simulink model "OMAP_ver_MIL10"  (R2018b)
settings: Solver=FixedStepDiscrete  StartTime=0.0  StopTime=10.0  FixedStep=0.01  RelTol=1e-3
undefined symbols (not defined in the file or in its folder): OMAP_Switch_EMS, OMAP_Switch_EPS, OMAP_Switch_ESC, OMAP_Switch_IC, OMAP_Switch_OTHER, TH_HMIClb_tiDgrdIconWarnHiDurT_C, TH_HMIClb_tiDgrdIconWarnLoDurT_C, TH_HMIClb_tiDgrdVocWarnDurT_C, TH_HMIClb_tiHndOffTxtWarnT_C, TH_HMIClb_tiHndOffVocWarnT_C, TH_HMIClb_tiSWALimFlgDetT_C, TH_HMIClb_tiTxtLimT_C
libraries: simulink x118
(part 1 of 9)
settings Model: Creator=许阁  LastModifiedBy=hj
settings OptimizationCC: BlockReduction=off  DefaultParameterBehavior=Inlined  DefaultUnderspecifiedDataType=single  EnhancedBackFolding=on  PassReuseOutputArgsAs=Individual arguments  ZeroExternalMemoryAtStartup=off  ZeroInternalMemoryAtStartup=off  OptimizeBlockOrder=speed  DifferentSizesBufferReuse=on  OptimizationCustomize=off
settings DebuggingCC: ParameterTunabilityLossMsg=error
settings SFSimCC: MATLABDynamicMemAlloc=off
settings RTWCC: SystemTargetFile=autosar.tlc  GenCodeOnly=on  TemplateMakefile=ert_default_tmf  Description=AUTOSAR  GenerateReport=on  IncludeHyperlinkInReport=on  LaunchReport=on  GenerateTraceInfo=on  GenerateTraceReport=on  GenerateTraceReportSl=on  GenerateTraceReportSf=on  GenerateTraceReportEml=on  GenerateCodeMetricsReport=on
settings CodeAppCC: ForceParamTrailComments=on  IgnoreCustomStorageClasses=off  OperatorAnnotations=on  SimulinkDataObjDesc=on  SFDataObjDesc=on  InsertBlockDesc=on
settings STFCustomTargetCC: TargetLangStandard=C99 (ISO)  MultiwordLength=256  ParMdlRefBuildCompliant=on  CompOptLevelCompliant=on  IncludeMdlTerminateFcn=off  CombineOutputUpdateFcns=on  SuppressErrorStatus=on  ERTCustomFileBanners=on  SupportNonFinite=off  SupportComplex=off  SupportContinuousTime=off  SupportNonInlinedSFcns=off  RemoveResetFunc=on  MATLABClassNameForMDSCustomization=Simulink.SoftwareTarget.ERTCustomization  AutosarCompliant=on  UseToolchainInfoCompliant=on  LookupTableObjectStructAxisOrder=2,1,3,4,...  LUTObjectStructOrderEvenSpacing=Size,Table,Breakpoints  SystemTargetFile=autosar.tlc
settings ERTTargetCC: TargetLangStandard=C99 (ISO)  ConcurrentExecutionCompliant=off  IncludeMdlTerminateFcn=off  SuppressErrorStatus=on  SupportNonFinite=off  SupportComplex=off  ModelStepFunctionPrototypeControlCompliant=off  CPPClassGenCompliant=off  AutosarCompliant=on  LookupTableObjectStructAxisOrder=2,1,3,4,...  LUTObjectStructOrderEvenSpacing=Size,Table,Breakpoints  GenerateASAP2=on  InlinedParameterPlacement=NonHierarchical  ERTCustomFileTemplate=example_file_process.tlc

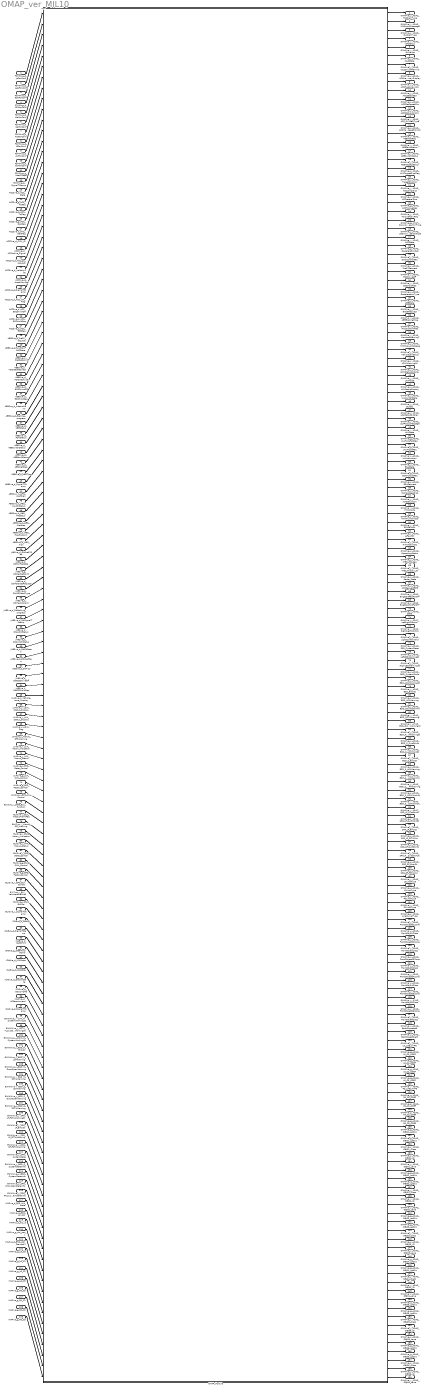
== system OMAP_ver_MIL10 ==
  FDMMve_d_JaFcnConf : Inport  OutDataTypeStr=UInt16  PortDimensions=1
  FDMMve_d_AebFcnConf : Inport  Port=2  OutDataTypeStr=UInt16  PortDimensions=1
  FDMMve_d_EsaFcnConf : Inport  Port=3  OutDataTypeStr=UInt16  PortDimensions=1
  FDMMve_d_ElkFcnConf : Inport  Port=4  OutDataTypeStr=UInt16  PortDimensions=1
  FDMMve_d_LkaFcnConf : Inport  Port=5  OutDataTypeStr=UInt16  PortDimensions=1
  FDMMve_d_IcaFcnConf : Inport  Port=6  OutDataTypeStr=UInt16  PortDimensions=1
  FDMMve_d_AccFcnConf : Inport  Port=7  OutDataTypeStr=UInt16  PortDimensions=1
  FDMMve_d_LfFcnConf : Inport  Port=8  OutDataTypeStr=UInt16  PortDimensions=1
  FDMMve_d_AlcFcnConf : Inport  Port=9  OutDataTypeStr=UInt16  PortDimensions=1
  FDMMve_d_EwFcnConf : Inport  Port=10  OutDataTypeStr=UInt16  PortDimensions=1
  FDMMve_g_Adas2Fapa : Inport  Port=11  OutDataTypeStr=UInt32  PortDimensions=1
  FDMMve_d_SignalTStamp : Inport  Port=12  OutDataTypeStr=UInt16  PortDimensions=1
  ACCSve_d_ACC_State : Inport  Port=13  OutDataTypeStr=UInt16  PortDimensions=1
  ACCSve_g_ACC_TqReq : Inport  Port=14  OutDataTypeStr=T_M_Nm_Float32  PortDimensions=1
  ACCSve_d_ACC_TqFlag : Inport  Port=15  OutDataTypeStr=UInt16  PortDimensions=1
  ACCSve_g_ACC_DecReq : Inport  Port=16  OutDataTypeStr=T_M_Nm_Float32  PortDimensions=1
  ACCSve_d_ACC_DecFlag : Inport  Port=17  OutDataTypeStr=UInt16  PortDimensions=1
  ACCSve_d_CIPV_ID : Inport  Port=18  OutDataTypeStr=UInt16  PortDimensions=1
  ACCSve_d_ACCActive_Signal : Inport  Port=19  OutDataTypeStr=UInt16  PortDimensions=1
  ACCSve_d_ACC_go_request : Inport  Port=20  OutDataTypeStr=UInt16  PortDimensions=1
  ACCSve_d_VelocitySet : Inport  Port=21  OutDataTypeStr=UInt16  PortDimensions=1
  ACCSve_d_HeadWaySet : Inport  Port=22  OutDataTypeStr=UInt16  PortDimensions=1
  ACCSve_d_SignalTStamp : Inport  Port=23  OutDataTypeStr=UInt16  PortDimensions=1
  ACCSve_d_ACC_ICA_Flag : Inport  Port=24  OutDataTypeStr=UInt16  PortDimensions=1
  ACCSve_d_ACC_ESCDriveOff : Inport  Port=25  OutDataTypeStr=UInt16  PortDimensions=1
  ACCSve_d_ACC_ESCHoldReq : Inport  Port=26  OutDataTypeStr=UInt16  PortDimensions=1
  ACCSve_d_ACC_EPBReq : Inport  Port=27  OutDataTypeStr=UInt16  PortDimensions=1
  AEBSve_d_Prefill_request : Inport  Port=28  OutDataTypeStr=UInt16  PortDimensions=1
  AEBSve_d_functionFARCState : Inport  Port=29  OutDataTypeStr=UInt16  PortDimensions=1
  AEBSve_g_DecSetpoint : Inport  Port=30  OutDataTypeStr=T_M_Nm_Float32  PortDimensions=1
  AEBSve_d_MDDdecRequest : Inport  Port=31  OutDataTypeStr=UInt16  PortDimensions=1
  AEBSve_d_MDDdecType : Inport  Port=32  OutDataTypeStr=UInt16  PortDimensions=1
  AEBSve_d_ESCDriveOff : Inport  Port=33  OutDataTypeStr=UInt16  PortDimensions=1
  AEBSve_d_ESCHoldReq : Inport  Port=34  OutDataTypeStr=UInt16  PortDimensions=1
  AEBSve_d_HapticAlarm : Inport  Port=35  OutDataTypeStr=UInt16  PortDimensions=1
  AEBSve_d_Braking_progress : Inport  Port=36  OutDataTypeStr=UInt16  PortDimensions=1
  AEBSve_d_AEBStatus : Inport  Port=37  OutDataTypeStr=UInt16  PortDimensions=1
  AEBSve_d_FCWStatus : Inport  Port=38  OutDataTypeStr=UInt16  PortDimensions=1
  AEBSve_d_AEBSwitchStatus : Inport  Port=39  OutDataTypeStr=UInt16  PortDimensions=1
  AEBSve_d_AEBFaultStatus : Inport  Port=40  OutDataTypeStr=UInt16  PortDimensions=1
  AEBSve_d_AEBAlertReq : Inport  Port=41  OutDataTypeStr=UInt16  PortDimensions=1
  AEBSve_d_AEBTips : Inport  Port=42  OutDataTypeStr=UInt16  PortDimensions=1
  AEBSve_d_SignalTStamp : Inport  Port=43  OutDataTypeStr=UInt16  PortDimensions=1
  AEBSve_d_JABS_AlertSign : Inport  Port=44  OutDataTypeStr=UInt16  PortDimensions=1
  AEBSve_d_JABS_SwitchStatus : Inport  Port=45  OutDataTypeStr=UInt16  PortDimensions=1
  AEBSve_d_JABS_FltStatus : Inport  Port=46  OutDataTypeStr=UInt16  PortDimensions=1
  AEBSve_d_JABS_AlertReq : Inport  Port=47  OutDataTypeStr=UInt16  PortDimensions=1
  AEBSve_d_JABS_HapticAlarm : Inport  Port=48  OutDataTypeStr=UInt16  PortDimensions=1
  AEBSve_d_JABS_Tips : Inport  Port=49  OutDataTypeStr=UInt16  PortDimensions=1
  JABSve_d_DbPrefillReq : Inport  Port=50  OutDataTypeStr=UInt16  PortDimensions=1
  JABSve_d_DbFunFARCSta : Inport  Port=51  OutDataTypeStr=UInt16  PortDimensions=1
  JABSve_g_DbDecSetpoint : Inport  Port=52  OutDataTypeStr=T_M_Nm_Float32  PortDimensions=1
  JABSve_d_DbMDDdecRequest : Inport  Port=53  OutDataTypeStr=UInt16  PortDimensions=1
  JABSve_d_DbMDDdecType : Inport  Port=54  OutDataTypeStr=UInt16  PortDimensions=1
  JABSve_d_DbHapticAlarm : Inport  Port=55  OutDataTypeStr=UInt16  PortDimensions=1
  JABSve_d_DbBraking_progress : Inport  Port=56  OutDataTypeStr=UInt16  PortDimensions=1
  JABSve_d_DbSignalTStamp : Inport  Port=57  OutDataTypeStr=UInt16  PortDimensions=1
  JABSve_d_DbJACWStatus : Inport  Port=58  OutDataTypeStr=UInt16  PortDimensions=1
  JABSve_d_DbSwitchStatus : Inport  Port=59  OutDataTypeStr=UInt16  PortDimensions=1
  JABSve_d_DbFltStatus : Inport  Port=60  OutDataTypeStr=UInt16  PortDimensions=1
  JABSve_d_DbAlertReq : Inport  Port=61  OutDataTypeStr=UInt16  PortDimensions=1
  JABSve_d_DbTips : Inport  Port=62  OutDataTypeStr=UInt16  PortDimensions=1
  JABSve_d_DbESCDriveOff : Inport  Port=63  OutDataTypeStr=UInt16  PortDimensions=1
  JABSve_d_DbESCHoldReq : Inport  Port=64  OutDataTypeStr=UInt16  PortDimensions=1
  LKASve_y_Vehicle_Lane_Display : Inport  Port=65  OutDataTypeStr=UInt8  PortDimensions=1
  LKASve_y_LDW_Status_Display : Inport  Port=66  OutDataTypeStr=UInt8  PortDimensions=1
  LKASve_y_LKA_Status_Display : Inport  Port=67  OutDataTypeStr=UInt8  PortDimensions=1
  LKASve_y_LDW_Flag : Inport  Port=68  OutDataTypeStr=UInt8  PortDimensions=1
  LKASve_y_Hands_Off_Warning : Inport  Port=69  OutDataTypeStr=UInt8  PortDimensions=1
  LKASve_y_LKA_Action_Indication : Inport  Port=70  OutDataTypeStr=UInt8  PortDimensions=1
  LKASve_y_HMI_Popup_Status : Inport  Port=71  OutDataTypeStr=UInt8  PortDimensions=1
  LKASve_y_EPS_State_Control : Inport  Port=72  OutDataTypeStr=UInt8  PortDimensions=1
  LKASve_g_LKA_SWA_Control : Inport  Port=73  OutDataTypeStr=T_M_Nm_Float32  PortDimensions=1
  LKASve_g_EPS_Factor_Control : Inport  Port=74  OutDataTypeStr=T_M_Nm_Float32  PortDimensions=1
  LKASve_y_EPS_LKA_Control : Inport  Port=75  OutDataTypeStr=UInt8  PortDimensions=1
  ELKSve_y_state_ELK_function : Inport  Port=76  OutDataTypeStr=UInt8  PortDimensions=1
  ELKSve_y_ELK_HapticAlarmReq : Inport  Port=77  OutDataTypeStr=UInt8  PortDimensions=1
  ELKSve_y_Hands_Off_Warning : Inport  Port=78  OutDataTypeStr=UInt8  PortDimensions=1
  ELKSve_y_ELK_Action_Indication : Inport  Port=79  OutDataTypeStr=UInt8  PortDimensions=1
  ELKSve_y_HMI_Popup_Status : Inport  Port=80  OutDataTypeStr=UInt8  PortDimensions=1
  ELKSve_y_EPS_State_Control : Inport  Port=81  OutDataTypeStr=UInt8  PortDimensions=1
  ELKSve_g_ELK_SWA_Control : Inport  Port=82  OutDataTypeStr=T_M_Nm_Float32  PortDimensions=1
  ELKSve_g_EPS_Factor_Control : Inport  Port=83  OutDataTypeStr=T_M_Nm_Float32  PortDimensions=1
  ELKSve_y_EPS_ELK_Control : Inport  Port=84  OutDataTypeStr=UInt8  PortDimensions=1
  ELKSve_y_ELK_VehicleLaneDisp : Inport  Port=85  OutDataTypeStr=UInt8  PortDimensions=1
  ELKSve_y_ELK_ELKSts : Inport  Port=86  OutDataTypeStr=UInt8  PortDimensions=1
  ELKSve_y_SignalTStamp : Inport  Port=87  OutDataTypeStr=UInt8  PortDimensions=1
  ICABva_d_PathQI : Inport  Port=88  OutDataTypeStr=UInt16  PortDimensions=6
  ICABve_d_SignalTStamp : Inport  Port=89  OutDataTypeStr=UInt16  PortDimensions=1
  ICABva_d_ICAB2HMI : Inport  Port=90  OutDataTypeStr=UInt16  PortDimensions=20
  ICABve_g_SteerAngleCmd : Inport  Port=91  OutDataTypeStr=T_M_Nm_Float32  PortDimensions=1
  ICABve_d_ICAMode : Inport  Port=92  OutDataTypeStr=UInt16  PortDimensions=1
  ICABve_d_ICAState : Inport  Port=93  OutDataTypeStr=UInt16  PortDimensions=1
  ICADva_d_DecionState : Inport  Port=94  OutDataTypeStr=UInt16  PortDimensions=10
  ICADva_d_DecionCMD : Inport  Port=95  OutDataTypeStr=UInt16  PortDimensions=10
  ICADva_d_LCRecommend : Inport  Port=96  OutDataTypeStr=UInt16  PortDimensions=10
  ICADve_d_SignalTStamp : Inport  Port=97  OutDataTypeStr=UInt16  PortDimensions=1
  EWWWve_y_LCW_M_SystemWorkingSt : Inport  Port=98  OutDataTypeStr=UInt8  PortDimensions=1
  EWWWve_y_RCTA_M_SystemWorkingSt : Inport  Port=99  OutDataTypeStr=UInt8  PortDimensions=1
  EWWWve_y_DOW_M_SystemWorkingSt : Inport  Port=100  OutDataTypeStr=UInt8  PortDimensions=1
  EWWWve_y_BSD_M_ErrorSt : Inport  Port=101  OutDataTypeStr=UInt8  PortDimensions=1
  EWWWve_y_BSD_M_LCAWarning : Inport  Port=102  OutDataTypeStr=UInt8  PortDimensions=1
  EWWWve_y_BSD_M_DoorOpenWarning : Inport  Port=103  OutDataTypeStr=UInt8  PortDimensions=1
  EWWWve_y_BSD_M_RCTAWarning : Inport  Port=104  OutDataTypeStr=UInt8  PortDimensions=1
  EWWWve_y_BSD_S_LCAWarning : Inport  Port=105  OutDataTypeStr=UInt8  PortDimensions=1
  EWWWve_y_BSD_S_DoorOpenWarning : Inport  Port=106  OutDataTypeStr=UInt8  PortDimensions=1
  EWWWve_y_BSD_S_RCTAWarning : Inport  Port=107  OutDataTypeStr=UInt8  PortDimensions=1
  EWWWve_y_SRR_LF_FCTAWorkingSt : Inport  Port=108  OutDataTypeStr=UInt8  PortDimensions=1
  EWWWve_y_SRR_LF_ErrorSt : Inport  Port=109  OutDataTypeStr=UInt8  PortDimensions=1
  EWWWve_y_SRR_LF_FCTAWarning : Inport  Port=110  OutDataTypeStr=UInt8  PortDimensions=1
  EWWWve_y_SRR_RF_FCTAWarning : Inport  Port=111  OutDataTypeStr=UInt8  PortDimensions=1
  EWWWve_y_SRR_SystemState : Inport  Port=112  OutDataTypeStr=UInt8  PortDimensions=1
  EWWWve_y_BSD_S_SystemStateInfo : Inport  Port=113  OutDataTypeStr=UInt8  PortDimensions=1
  EWWWve_y_BSD_SystemStateInfo : Inport  Port=114  OutDataTypeStr=UInt8  PortDimensions=1
  EWWWve_y_SRR_LF_SystemStateInfo : Inport  Port=115  OutDataTypeStr=UInt8  PortDimensions=1
  EWWWve_y_SRR_RF_SystemStateInfo : Inport  Port=116  OutDataTypeStr=UInt8  PortDimensions=1
  IMAPve_d_EPS_LKA_State : Inport  Port=117  OutDataTypeStr=UInt16  PortDimensions=1
  IMAPve_g_ESC_LonAcc : Inport  Port=118  OutDataTypeStr=T_M_Nm_Float32  PortDimensions=1
  IMAPva_d_obj_id : Inport  Port=119  OutDataTypeStr=UInt16  PortDimensions=40
  IMAPva_g_obj_pos_x : Inport  Port=120  OutDataTypeStr=T_M_Nm_Float32  PortDimensions=40
  IMAPve_d_ESC_Veh_Standstill : Inport  Port=121  OutDataTypeStr=UInt16  PortDimensions=1
  IMAPve_g_L0_C0 : Inport  Port=122  OutDataTypeStr=T_M_Nm_Float32  PortDimensions=1
  IMAPve_g_L0_C1 : Inport  Port=123  OutDataTypeStr=T_M_Nm_Float32  PortDimensions=1
  IMAPve_g_L0_C2 : Inport  Port=124  OutDataTypeStr=T_M_Nm_Float32  PortDimensions=1
  IMAPve_g_L0_C3 : Inport  Port=125  OutDataTypeStr=T_M_Nm_Float32  PortDimensions=1
  IMAPve_g_R0_C0 : Inport  Port=126  OutDataTypeStr=T_M_Nm_Float32  PortDimensions=1
  IMAPve_g_R0_C1 : Inport  Port=127  OutDataTypeStr=T_M_Nm_Float32  PortDimensions=1
  IMAPve_g_R0_C2 : Inport  Port=128  OutDataTypeStr=T_M_Nm_Float32  PortDimensions=1
  IMAPve_g_R0_C3 : Inport  Port=129  OutDataTypeStr=T_M_Nm_Float32  PortDimensions=1
  OMAP_Module : Subsystem  TreatAsAtomicUnit=on
  OMAPve_y_ADAS_TSRSignType : Outport  OutDataTypeStr=UInt8  PortDimensions=1
  OMAPve_y_ADAS_ISAPopupMessage : Outport  Port=2  OutDataTypeStr=UInt8  PortDimensions=1
  OMAPve_y_ADAS_ISASignType : Outport  Port=3  OutDataTypeStr=UInt8  PortDimensions=1
  OMAPve_y_ADAS_ISAStatus : Outport  Port=4  OutDataTypeStr=UInt8  PortDimensions=1
  OMAPve_y_ADAS_ISAValue : Outport  Port=5  OutDataTypeStr=UInt8  PortDimensions=1
  OMAPve_y_ADAS_ISLCState : Outport  Port=6  OutDataTypeStr=UInt8  PortDimensions=1
  OMAPve_y_ADAS_ISLCDriverRemind : Outport  Port=7  OutDataTypeStr=UInt8  PortDimensions=1
  OMAPve_y_ADAS_ACCHeadwayDisplay : Outport  Port=8  OutDataTypeStr=UInt8  PortDimensions=1
  OMAPve_y_ADAS_ACCHeadwayIcon : Outport  Port=9  OutDataTypeStr=UInt8  PortDimensions=1
  OMAPve_y_ADAS_ACCSetSpeed : Outport  Port=10  OutDataTypeStr=UInt8  PortDimensions=1
  OMAPve_y_ADAS_ACCSetSpeedDis : Outport  Port=11  OutDataTypeStr=UInt8  PortDimensions=1
  OMAPve_y_ADAS_ACCStatusIconDis : Outport  Port=12  OutDataTypeStr=UInt8  PortDimensions=1
  OMAPve_y_ADAS_ACC_RVVReqType : Outport  Port=13  OutDataTypeStr=UInt8  PortDimensions=1
  OMAPve_y_ADAS_ACCMessagePrompt : Outport  Port=14  OutDataTypeStr=UInt8  PortDimensions=1
  OMAPve_y_ADAS_AEBAlertReq : Outport  Port=15  OutDataTypeStr=UInt8  PortDimensions=1
  OMAPve_y_ADAS_AEBFaultStatus : Outport  Port=16  OutDataTypeStr=UInt8  PortDimensions=1
  OMAPve_y_ADAS_AEBSwitchStatus : Outport  Port=17  OutDataTypeStr=UInt8  PortDimensions=1
  OMAPve_y_ADAS_AEBMassageDisp : Outport  Port=18  OutDataTypeStr=UInt8  PortDimensions=1
  OMAPve_y_ADAS_HMITargetDispFlag : Outport  Port=19  OutDataTypeStr=UInt8  PortDimensions=1
  OMAPve_y_ADAS_TargetPosition : Outport  Port=20  OutDataTypeStr=UInt8  PortDimensions=1
  OMAPve_y_ADAS_ACCLongiDist : Outport  Port=21  OutDataTypeStr=UInt8  PortDimensions=1
  OMAPve_y_ADAS_ACCLateralDist : Outport  Port=22  OutDataTypeStr=SInt8  PortDimensions=1
  OMAPve_g_ADAS_ACCTorqueReq : Outport  Port=23  OutDataTypeStr=T_M_Nm_Float32  PortDimensions=1
  OMAPve_y_ADAS_TorqueActivReq : Outport  Port=24  OutDataTypeStr=UInt8  PortDimensions=1
  OMAPve_g_ADAS_DownorUpGearMinTime : Outport  Port=25  OutDataTypeStr=T_M_Nm_Float32  PortDimensions=1
  OMAPve_y_ADAS_UpDownGearChange : Outport  Port=26  OutDataTypeStr=UInt8  PortDimensions=1
  OMAPve_y_ADAS_ACCState : Outport  Port=27  OutDataTypeStr=UInt8  PortDimensions=1
  OMAPve_g_ADAS_DecelerationSet : Outport  Port=28  OutDataTypeStr=T_M_Nm_Float32  PortDimensions=1
  OMAPve_y_ADAS_DeclControlReq : Outport  Port=29  OutDataTypeStr=UInt8  PortDimensions=1
  OMAPve_y_ADAS_PrefillRequest : Outport  Port=30  OutDataTypeStr=UInt8  PortDimensions=1
  OMAPve_y_ADAS_ESCDriveOff : Outport  Port=31  OutDataTypeStr=UInt8  PortDimensions=1
  OMAPve_y_ADAS_ESCHoldReq : Outport  Port=32  OutDataTypeStr=UInt8  PortDimensions=1
  OMAPve_y_ADAS_DecelerationType : Outport  Port=33  OutDataTypeStr=UInt8  PortDimensions=1
  OMAPve_y_ADAS_AEBState : Outport  Port=34  OutDataTypeStr=UInt8  PortDimensions=1
  OMAPve_y_ADAS_BrakeRequest : Outport  Port=35  OutDataTypeStr=UInt8  PortDimensions=1
  OMAPve_y_ADAS_AEBBrakingProg : Outport  Port=36  OutDataTypeStr=UInt8  PortDimensions=1
  OMAPve_y_ADAS_HapticAlarmReq : Outport  Port=37  OutDataTypeStr=UInt8  PortDimensions=1
  OMAPve_y_ADAS_Handsoffwarning : Outport  Port=38  OutDataTypeStr=UInt8  PortDimensions=1
  OMAPve_y_ADAS_HMIPopupMassage : Outport  Port=39  OutDataTypeStr=UInt8  PortDimensions=1
  OMAPve_y_ADAS_VehicleLaneDisp : Outport  Port=40  OutDataTypeStr=UInt8  PortDimensions=1
  OMAPve_y_ADAS_LDWWarningSt : Outport  Port=41  OutDataTypeStr=UInt8  PortDimensions=1
  OMAPve_y_ADAS_LDWStatusDisplay : Outport  Port=42  OutDataTypeStr=UInt8  PortDimensions=1
  OMAPve_y_ADAS_LKAMode : Outport  Port=43  OutDataTypeStr=UInt8  PortDimensions=1
  OMAPve_y_ADAS_LKAStatusDisplay : Outport  Port=44  OutDataTypeStr=UInt8  PortDimensions=1
  OMAPve_y_ADAS_LKASwitchState : Outport  Port=45  OutDataTypeStr=UInt8  PortDimensions=1
  OMAPve_y_ADAS_ELKSts : Outport  Port=46  OutDataTypeStr=UInt8  PortDimensions=1
  OMAPve_y_ADAS_LCAStatusDisplay : Outport  Port=47  OutDataTypeStr=UInt8  PortDimensions=1
  OMAPve_y_ADAS_LCAPopupMessage : Outport  Port=48  OutDataTypeStr=UInt8  PortDimensions=1
  OMAPve_y_ADAS_LKAState : Outport  Port=49  OutDataTypeStr=UInt8  PortDimensions=1
  OMAPve_g_ADAS_LKATorqFactReq : Outport  Port=50  OutDataTypeStr=T_M_Nm_Float32  PortDimensions=1
  OMAPve_g_ADAS_LKAAngleReq : Outport  Port=51  OutDataTypeStr=T_M_Nm_Float32  PortDimensions=1
  OMAPve_y_ADAS_LKAActivation : Outport  Port=52  OutDataTypeStr=UInt8  PortDimensions=1
  OMAPve_y_ADAS_ESAState : Outport  Port=53  OutDataTypeStr=UInt8  PortDimensions=1
  OMAPve_g_ADAS_ESATorqueReq : Outport  Port=54  OutDataTypeStr=T_M_Nm_Float32  PortDimensions=1
  OMAPve_y_ADAS_ESARequest : Outport  Port=55  OutDataTypeStr=UInt8  PortDimensions=1
  OMAPve_y_ADAS_ICAMassageDisp : Outport  Port=56  OutDataTypeStr=UInt8  PortDimensions=1
  OMAPve_y_ADAS_ICAStatusIcon : Outport  Port=57  OutDataTypeStr=UInt8  PortDimensions=1
  OMAPve_y_ADAS_HWAMode : Outport  Port=58  OutDataTypeStr=UInt8  PortDimensions=1
  OMAPve_y_ADAS_HWATurnOnIdctr : Outport  Port=59  OutDataTypeStr=UInt8  PortDimensions=1
  OMAPve_y_ADAS_ESAFaultSt : Outport  Port=60  OutDataTypeStr=UInt8  PortDimensions=1
  OMAPve_y_ADAS_JAFaultSt : Outport  Port=61  OutDataTypeStr=UInt8  PortDimensions=1
  OMAPve_y_ADAS_HWAActionSts : Outport  Port=62  OutDataTypeStr=UInt8  PortDimensions=1
  OMAPve_y_ADAS_OperatingStatus : Outport  Port=63  OutDataTypeStr=UInt8  PortDimensions=1
  OMAPve_y_ADAS_IHBC_HB_Req : Outport  Port=64  OutDataTypeStr=UInt8  PortDimensions=1
  OMAPve_y_ADAS_IHBC_Fuction_St : Outport  Port=65  OutDataTypeStr=UInt8  PortDimensions=1
  OMAPve_y_ADAS_Radar_State : Outport  Port=66  OutDataTypeStr=UInt8  PortDimensions=1
  OMAPve_y_ADAS_ACCRequestEPB : Outport  Port=67  OutDataTypeStr=UInt8  PortDimensions=1
  OMAPve_y_ADAS_EngStartReqForSTT : Outport  Port=68  OutDataTypeStr=UInt8  PortDimensions=1
  OMAPve_y_ADAS_EngStopPmtForSTT : Outport  Port=69  OutDataTypeStr=UInt8  PortDimensions=1
  OMAPve_y_ADAS_State : Outport  Port=70  OutDataTypeStr=UInt8  PortDimensions=1
  OMAPve_y_ADAS_LetfLigthControl : Outport  Port=71  OutDataTypeStr=UInt8  PortDimensions=1
  OMAPve_y_ADAS_RightLigthControl : Outport  Port=72  OutDataTypeStr=UInt8  PortDimensions=1
  OMAPve_y_ADAS_LightControlValid : Outport  Port=73  OutDataTypeStr=UInt8  PortDimensions=1
  OMAPve_y_ADAS_SRR_SystemState : Outport  Port=74  OutDataTypeStr=UInt8  PortDimensions=1
  OMAPve_y_ADAS_LeftLEDWarningSt : Outport  Port=75  OutDataTypeStr=UInt8  PortDimensions=1
  OMAPve_y_ADAS_RighrLEDWarningSt : Outport  Port=76  OutDataTypeStr=UInt8  PortDimensions=1
  OMAPve_y_ADAS_BSD_SystemStInfo : Outport  Port=77  OutDataTypeStr=UInt8  PortDimensions=1
  OMAPve_y_ADAS_BSD_LCWWorkingSt : Outport  Port=78  OutDataTypeStr=UInt8  PortDimensions=1
  OMAPve_y_ADAS_BSD_ErrorSt : Outport  Port=79  OutDataTypeStr=UInt8  PortDimensions=1
  OMAPve_y_ADAS_BSD_LCAWarning : Outport  Port=80  OutDataTypeStr=UInt8  PortDimensions=1
  OMAPve_y_ADAS_BSD_DoorOpenWrn : Outport  Port=81  OutDataTypeStr=UInt8  PortDimensions=1
  OMAPve_y_ADAS_BSD_RCTAWarning : Outport  Port=82  OutDataTypeStr=UInt8  PortDimensions=1
  OMAPve_y_ADAS_BSD_DOWWorkingSt : Outport  Port=83  OutDataTypeStr=UInt8  PortDimensions=1
  OMAPve_y_ADAS_BSD_RCTAWorkingSt : Outport  Port=84  OutDataTypeStr=UInt8  PortDimensions=1
  OMAPve_y_ADAS_BSD_S_SystStInfo : Outport  Port=85  OutDataTypeStr=UInt8  PortDimensions=1
  OMAPve_y_ADAS_BSD_S_LCWWorkSt : Outport  Port=86  OutDataTypeStr=UInt8  PortDimensions=1
  OMAPve_y_ADAS_BSD_S_ErrorSt : Outport  Port=87  OutDataTypeStr=UInt8  PortDimensions=1
  OMAPve_y_ADAS_BSD_S_LCAWarning : Outport  Port=88  OutDataTypeStr=UInt8  PortDimensions=1
  OMAPve_y_ADAS_BSD_S_DoorOpenWrn : Outport  Port=89  OutDataTypeStr=UInt8  PortDimensions=1
  OMAPve_y_ADAS_BSD_S_RCTAWarning : Outport  Port=90  OutDataTypeStr=UInt8  PortDimensions=1
  OMAPve_y_ADAS_BSD_S_DOWWorkSt : Outport  Port=91  OutDataTypeStr=UInt8  PortDimensions=1
  OMAPve_y_ADAS_BSD_S_RCTAWorkSt : Outport  Port=92  OutDataTypeStr=UInt8  PortDimensions=1
  OMAPve_y_ADAS_SRR_LF_SystStInfo : Outport  Port=93  OutDataTypeStr=UInt8  PortDimensions=1
  OMAPve_y_ADAS_SRR_LF_SystWorkSt : Outport  Port=94  OutDataTypeStr=UInt8  PortDimensions=1
  OMAPve_y_ADAS_SRR_LF_ErrorSt : Outport  Port=95  OutDataTypeStr=UInt8  PortDimensions=1
  OMAPve_y_ADAS_SRR_LF_FCTAWrn : Outport  Port=96  OutDataTypeStr=UInt8  PortDimensions=1
  OMAPve_y_ADAS_SRR_RF_SystStInfo : Outport  Port=97  OutDataTypeStr=UInt8  PortDimensions=1
  OMAPve_y_ADAS_SRR_RF_SystWorkSt : Outport  Port=98  OutDataTypeStr=UInt8  PortDimensions=1
  OMAPve_y_ADAS_SRR_RF_ErrorSt : Outport  Port=99  OutDataTypeStr=UInt8  PortDimensions=1
  OMAPve_y_ADAS_SRR_RF_FCTAWrn : Outport  Port=100  OutDataTypeStr=UInt8  PortDimensions=1
  OMAPve_y_ADAS_L0LineType : Outport  Port=101  OutDataTypeStr=UInt8  PortDimensions=1
  OMAPve_y_ADAS_L1LineType : Outport  Port=102  OutDataTypeStr=UInt8  PortDimensions=1
  OMAPve_y_ADAS_R0LineType : Outport  Port=103  OutDataTypeStr=UInt8  PortDimensions=1
  OMAPve_y_ADAS_R1LineType : Outport  Port=104  OutDataTypeStr=UInt8  PortDimensions=1
  OMAPve_y_ADAS_LineCurveType : Outport  Port=105  OutDataTypeStr=UInt8  PortDimensions=1
  OMAPve_y_ADAS_FrontObject01Zone : Outport  Port=106  OutDataTypeStr=UInt8  PortDimensions=1
  OMAPve_y_ADAS_FrontObj01Class : Outport  Port=107  OutDataTypeStr=UInt8  PortDimensions=1
  OMAPve_y_ADAS_FrontObject02Zone : Outport  Port=108  OutDataTypeStr=UInt8  PortDimensions=1
  OMAPve_y_ADAS_FrontObj02Class : Outport  Port=109  OutDataTypeStr=UInt8  PortDimensions=1
  OMAPve_y_ADAS_FrontObject03Zone : Outport  Port=110  OutDataTypeStr=UInt8  PortDimensions=1
  OMAPve_y_ADAS_FrontObj03Class : Outport  Port=111  OutDataTypeStr=UInt8  PortDimensions=1
  OMAPve_y_ADAS_FrontObject04Zone : Outport  Port=112  OutDataTypeStr=UInt8  PortDimensions=1
  OMAPve_y_ADAS_FrontObj04Class : Outport  Port=113  OutDataTypeStr=UInt8  PortDimensions=1
  OMAPve_y_ADAS_FrontObject05Zone : Outport  Port=114  OutDataTypeStr=UInt8  PortDimensions=1
  OMAPve_y_ADAS_FrontObj05Class : Outport  Port=115  OutDataTypeStr=UInt8  PortDimensions=1
  OMAPve_y_ADAS_FrontObject06Zone : Outport  Port=116  OutDataTypeStr=UInt8  PortDimensions=1
  OMAPve_y_ADAS_FrontObj06Class : Outport  Port=117  OutDataTypeStr=UInt8  PortDimensions=1
  OMAPve_y_ADAS_BackObjectLeft : Outport  Port=118  OutDataTypeStr=UInt8  PortDimensions=1
  OMAPve_y_ADAS_BackObjectRight : Outport  Port=119  OutDataTypeStr=UInt8  PortDimensions=1
  OMAPve_y_ADAS_L0_LINE_TYPE : Outport  Port=120  OutDataTypeStr=UInt8  PortDimensions=1
  OMAPve_g_ADAS_L0_C0_COEF : Outport  Port=121  OutDataTypeStr=T_M_Nm_Float32  PortDimensions=1
  OMAPve_g_ADAS_L0_C1_COEF : Outport  Port=122  OutDataTypeStr=T_M_Nm_Float32  PortDimensions=1
  OMAPve_g_ADAS_L0_C2_COEF : Outport  Port=123  OutDataTypeStr=T_M_Nm_Float32  PortDimensions=1
  OMAPve_g_ADAS_L0_C3_COEF : Outport  Port=124  OutDataTypeStr=T_M_Nm_Float32  PortDimensions=1
  OMAPve_y_ADAS_R0_LINE_TYPE : Outport  Port=125  OutDataTypeStr=UInt8  PortDimensions=1
  OMAPve_g_ADAS_R0_C0_COEF : Outport  Port=126  OutDataTypeStr=T_M_Nm_Float32  PortDimensions=1
  OMAPve_g_ADAS_R0_C1_COEF : Outport  Port=127  OutDataTypeStr=T_M_Nm_Float32  PortDimensions=1
  OMAPve_g_ADAS_R0_C2_COEF : Outport  Port=128  OutDataTypeStr=T_M_Nm_Float32  PortDimensions=1
  OMAPve_g_ADAS_R0_C3_COEF : Outport  Port=129  OutDataTypeStr=T_M_Nm_Float32  PortDimensions=1
  OMAPve_g_ADAS_OBJ01_LatDis : Outport  Port=130  OutDataTypeStr=T_M_Nm_Float32  PortDimensions=1
  OMAPve_g_ADAS_OBJ01_LgtDis : Outport  Port=131  OutDataTypeStr=T_M_Nm_Float32  PortDimensions=1
  OMAPve_y_ADAS_OBJ01_Class : Outport  Port=132  OutDataTypeStr=UInt8  PortDimensions=1
  OMAPve_y_ADAS_OBJ01_ID : Outport  Port=133  OutDataTypeStr=UInt8  PortDimensions=1
  OMAPve_y_ADAS_OBJ01_Lane : Outport  Port=134  OutDataTypeStr=UInt8  PortDimensions=1
  OMAPve_g_ADAS_OBJ02_LatDis : Outport  Port=135  OutDataTypeStr=T_M_Nm_Float32  PortDimensions=1
  OMAPve_g_ADAS_OBJ02_LgtDis : Outport  Port=136  OutDataTypeStr=T_M_Nm_Float32  PortDimensions=1
  OMAPve_y_ADAS_OBJ02_Class : Outport  Port=137  OutDataTypeStr=UInt8  PortDimensions=1
  OMAPve_y_ADAS_OBJ02_ID : Outport  Port=138  OutDataTypeStr=UInt8  PortDimensions=1
  OMAPve_y_ADAS_OBJ02_Lane : Outport  Port=139  OutDataTypeStr=UInt8  PortDimensions=1
  OMAPve_g_ADAS_OBJ03_LatDis : Outport  Port=140  OutDataTypeStr=T_M_Nm_Float32  PortDimensions=1
  OMAPve_g_ADAS_OBJ03_LgtDis : Outport  Port=141  OutDataTypeStr=T_M_Nm_Float32  PortDimensions=1
  OMAPve_y_ADAS_OBJ03_Class : Outport  Port=142  OutDataTypeStr=UInt8  PortDimensions=1
  OMAPve_y_ADAS_OBJ03_ID : Outport  Port=143  OutDataTypeStr=UInt8  PortDimensions=1
  OMAPve_y_ADAS_OBJ03_Lane : Outport  Port=144  OutDataTypeStr=UInt8  PortDimensions=1
  OMAPve_g_ADAS_OBJ04_LatDis : Outport  Port=145  OutDataTypeStr=T_M_Nm_Float32  PortDimensions=1
  OMAPve_g_ADAS_OBJ04_LgtDis : Outport  Port=146  OutDataTypeStr=T_M_Nm_Float32  PortDimensions=1
  OMAPve_y_ADAS_OBJ04_Class : Outport  Port=147  OutDataTypeStr=UInt8  PortDimensions=1
  OMAPve_y_ADAS_OBJ04_ID : Outport  Port=148  OutDataTypeStr=UInt8  PortDimensions=1
  OMAPve_y_ADAS_OBJ04_Lane : Outport  Port=149  OutDataTypeStr=UInt8  PortDimensions=1
  OMAPve_g_ADAS_OBJ05_LatDis : Outport  Port=150  OutDataTypeStr=T_M_Nm_Float32  PortDimensions=1
  OMAPve_g_ADAS_OBJ05_LgtDis : Outport  Port=151  OutDataTypeStr=T_M_Nm_Float32  PortDimensions=1
  OMAPve_y_ADAS_OBJ05_Class : Outport  Port=152  OutDataTypeStr=UInt8  PortDimensions=1
  OMAPve_y_ADAS_OBJ05_ID : Outport  Port=153  OutDataTypeStr=UInt8  PortDimensions=1
  OMAPve_y_ADAS_OBJ05_Lane : Outport  Port=154  OutDataTypeStr=UInt8  PortDimensions=1
  OMAPve_g_ADAS_OBJ06_LatDis : Outport  Port=155  OutDataTypeStr=T_M_Nm_Float32  PortDimensions=1
  OMAPve_g_ADAS_OBJ06_LgtDis : Outport  Port=156  OutDataTypeStr=T_M_Nm_Float32  PortDimensions=1
  OMAPve_y_ADAS_OBJ06_Class : Outport  Port=157  OutDataTypeStr=UInt8  PortDimensions=1
  OMAPve_y_ADAS_OBJ06_ID : Outport  Port=158  OutDataTypeStr=UInt8  PortDimensions=1
  OMAPve_y_ADAS_OBJ06_Lane : Outport  Port=159  OutDataTypeStr=UInt8  PortDimensions=1
  wires:
  ACCSve_d_ACC_State/1 -> OMAP_Module/13(ACCSve_d_ACC_State)
  OMAP_Module/134(OMAPve_y_ADAS_OBJ01_Lane) -> OMAPve_y_ADAS_OBJ01_Lane/1
  OMAP_Module/42(OMAPve_y_ADAS_LDWStatusDisplay) -> OMAPve_y_ADAS_LDWStatusDisplay/1
  OMAP_Module/118(OMAPve_y_ADAS_BackObjectLeft) -> OMAPve_y_ADAS_BackObjectLeft/1
  FDMMve_d_SignalTStamp/1 -> OMAP_Module/12(FDMMve_d_SignalTStamp)
  AEBSve_d_JABS_SwitchStatus/1 -> OMAP_Module/45(AEBSve_d_JABS_SwitchStatus)
  OMAP_Module/113(OMAPve_y_ADAS_FrontObj04Class) -> OMAPve_y_ADAS_FrontObj04Class/1
  EWWWve_y_BSD_S_LCAWarning/1 -> OMAP_Module/105(EWWWve_y_BSD_S_LCAWarning)
  OMAP_Module/44(OMAPve_y_ADAS_LKAStatusDisplay) -> OMAPve_y_ADAS_LKAStatusDisplay/1
  OMAP_Module/79(OMAPve_y_ADAS_BSD_ErrorSt) -> OMAPve_y_ADAS_BSD_ErrorSt/1
  ICADva_d_DecionState/1 -> OMAP_Module/94(ICADva_d_DecionState)
  FDMMve_d_IcaFcnConf/1 -> OMAP_Module/6(FDMMve_d_IcaFcnConf)
  OMAP_Module/90(OMAPve_y_ADAS_BSD_S_RCTAWarning) -> OMAPve_y_ADAS_BSD_S_RCTAWarning/1
  OMAP_Module/148(OMAPve_y_ADAS_OBJ04_ID) -> OMAPve_y_ADAS_OBJ04_ID/1
  OMAP_Module/65(OMAPve_y_ADAS_IHBC_Fuction_St) -> OMAPve_y_ADAS_IHBC_Fuction_St/1
  OMAP_Module/111(OMAPve_y_ADAS_FrontObj03Class) -> OMAPve_y_ADAS_FrontObj03Class/1
  JABSve_d_DbESCDriveOff/1 -> OMAP_Module/63(JABSve_d_DbESCDriveOff)
  ICABva_d_PathQI/1 -> OMAP_Module/88(ICABva_d_PathQI)
  FDMMve_d_EsaFcnConf/1 -> OMAP_Module/3(FDMMve_d_EsaFcnConf)
  OMAP_Module/78(OMAPve_y_ADAS_BSD_LCWWorkingSt) -> OMAPve_y_ADAS_BSD_LCWWorkingSt/1
  OMAP_Module/63(OMAPve_y_ADAS_OperatingStatus) -> OMAPve_y_ADAS_OperatingStatus/1
  IMAPve_g_L0_C0/1 -> OMAP_Module/122(IMAPve_g_L0_C0)
  OMAP_Module/156(OMAPve_g_ADAS_OBJ06_LgtDis) -> OMAPve_g_ADAS_OBJ06_LgtDis/1
  JABSve_d_DbBraking_progress/1 -> OMAP_Module/56(JABSve_d_DbBraking_progress)
  EWWWve_y_DOW_M_SystemWorkingSt/1 -> OMAP_Module/100(EWWWve_y_DOW_M_SystemWorkingSt)
  OMAP_Module/72(OMAPve_y_ADAS_RightLigthControl) -> OMAPve_y_ADAS_RightLigthControl/1
  EWWWve_y_SRR_LF_ErrorSt/1 -> OMAP_Module/109(EWWWve_y_SRR_LF_ErrorSt)
  IMAPve_g_L0_C3/1 -> OMAP_Module/125(IMAPve_g_L0_C3)
  ACCSve_d_ACC_EPBReq/1 -> OMAP_Module/27(ACCSve_d_ACC_EPBReq)
  ACCSve_d_CIPV_ID/1 -> OMAP_Module/18(ACCSve_d_CIPV_ID)
  AEBSve_d_ESCDriveOff/1 -> OMAP_Module/33(AEBSve_d_ESCDriveOff)
  AEBSve_d_JABS_AlertReq/1 -> OMAP_Module/47(AEBSve_d_JABS_AlertReq)
  OMAP_Module/2(OMAPve_y_ADAS_ISAPopupMessage) -> OMAPve_y_ADAS_ISAPopupMessage/1
  FDMMve_d_JaFcnConf/1 -> OMAP_Module/1(FDMMve_d_JaFcnConf)
  AEBSve_g_DecSetpoint/1 -> OMAP_Module/30(AEBSve_g_DecSetpoint)
  OMAP_Module/122(OMAPve_g_ADAS_L0_C1_COEF) -> OMAPve_g_ADAS_L0_C1_COEF/1
  OMAP_Module/82(OMAPve_y_ADAS_BSD_RCTAWarning) -> OMAPve_y_ADAS_BSD_RCTAWarning/1
  IMAPve_g_R0_C3/1 -> OMAP_Module/129(IMAPve_g_R0_C3)
  ACCSve_d_ACC_ESCHoldReq/1 -> OMAP_Module/26(ACCSve_d_ACC_ESCHoldReq)
  OMAP_Module/141(OMAPve_g_ADAS_OBJ03_LgtDis) -> OMAPve_g_ADAS_OBJ03_LgtDis/1
  OMAP_Module/66(OMAPve_y_ADAS_Radar_State) -> OMAPve_y_ADAS_Radar_State/1
  IMAPve_g_L0_C2/1 -> OMAP_Module/124(IMAPve_g_L0_C2)
  OMAP_Module/69(OMAPve_y_ADAS_EngStopPmtForSTT) -> OMAPve_y_ADAS_EngStopPmtForSTT/1
  IMAPva_g_obj_pos_x/1 -> OMAP_Module/120(IMAPva_g_obj_pos_x)
  OMAP_Module/110(OMAPve_y_ADAS_FrontObject03Zone) -> OMAPve_y_ADAS_FrontObject03Zone/1
  OMAP_Module/127(OMAPve_g_ADAS_R0_C1_COEF) -> OMAPve_g_ADAS_R0_C1_COEF/1
  ICABve_d_ICAState/1 -> OMAP_Module/93(ICABve_d_ICAState)
  LKASve_g_LKA_SWA_Control/1 -> OMAP_Module/73(LKASve_g_LKA_SWA_Control)
  AEBSve_d_FCWStatus/1 -> OMAP_Module/38(AEBSve_d_FCWStatus)
  ACCSve_d_HeadWaySet/1 -> OMAP_Module/22(ACCSve_d_HeadWaySet)
  OMAP_Module/6(OMAPve_y_ADAS_ISLCState) -> OMAPve_y_ADAS_ISLCState/1
  FDMMve_d_ElkFcnConf/1 -> OMAP_Module/4(FDMMve_d_ElkFcnConf)
  OMAP_Module/33(OMAPve_y_ADAS_DecelerationType) -> OMAPve_y_ADAS_DecelerationType/1
  IMAPve_d_EPS_LKA_State/1 -> OMAP_Module/117(IMAPve_d_EPS_LKA_State)
  OMAP_Module/145(OMAPve_g_ADAS_OBJ04_LatDis) -> OMAPve_g_ADAS_OBJ04_LatDis/1
  OMAP_Module/85(OMAPve_y_ADAS_BSD_S_SystStInfo) -> OMAPve_y_ADAS_BSD_S_SystStInfo/1
  OMAP_Module/8(OMAPve_y_ADAS_ACCHeadwayDisplay) -> OMAPve_y_ADAS_ACCHeadwayDisplay/1
  OMAP_Module/31(OMAPve_y_ADAS_ESCDriveOff) -> OMAPve_y_ADAS_ESCDriveOff/1
  OMAP_Module/117(OMAPve_y_ADAS_FrontObj06Class) -> OMAPve_y_ADAS_FrontObj06Class/1
  IMAPve_g_L0_C1/1 -> OMAP_Module/123(IMAPve_g_L0_C1)
  OMAP_Module/119(OMAPve_y_ADAS_BackObjectRight) -> OMAPve_y_ADAS_BackObjectRight/1
  OMAP_Module/36(OMAPve_y_ADAS_AEBBrakingProg) -> OMAPve_y_ADAS_AEBBrakingProg/1
  OMAP_Module/132(OMAPve_y_ADAS_OBJ01_Class) -> OMAPve_y_ADAS_OBJ01_Class/1
  OMAP_Module/152(OMAPve_y_ADAS_OBJ05_Class) -> OMAPve_y_ADAS_OBJ05_Class/1
  OMAP_Module/105(OMAPve_y_ADAS_LineCurveType) -> OMAPve_y_ADAS_LineCurveType/1
  ACCSve_d_VelocitySet/1 -> OMAP_Module/21(ACCSve_d_VelocitySet)
  ELKSve_y_SignalTStamp/1 -> OMAP_Module/87(ELKSve_y_SignalTStamp)
  OMAP_Module/99(OMAPve_y_ADAS_SRR_RF_ErrorSt) -> OMAPve_y_ADAS_SRR_RF_ErrorSt/1
  OMAP_Module/58(OMAPve_y_ADAS_HWAMode) -> OMAPve_y_ADAS_HWAMode/1
  OMAP_Module/140(OMAPve_g_ADAS_OBJ03_LatDis) -> OMAPve_g_ADAS_OBJ03_LatDis/1
  OMAP_Module/104(OMAPve_y_ADAS_R1LineType) -> OMAPve_y_ADAS_R1LineType/1
  OMAP_Module/70(OMAPve_y_ADAS_State) -> OMAPve_y_ADAS_State/1
  OMAP_Module/158(OMAPve_y_ADAS_OBJ06_ID) -> OMAPve_y_ADAS_OBJ06_ID/1
  OMAP_Module/155(OMAPve_g_ADAS_OBJ06_LatDis) -> OMAPve_g_ADAS_OBJ06_LatDis/1
  OMAP_Module/84(OMAPve_y_ADAS_BSD_RCTAWorkingSt) -> OMAPve_y_ADAS_BSD_RCTAWorkingSt/1
  JABSve_d_DbMDDdecType/1 -> OMAP_Module/54(JABSve_d_DbMDDdecType)
  EWWWve_y_SRR_RF_SystemStateInfo/1 -> OMAP_Module/116(EWWWve_y_SRR_RF_SystemStateInfo)
  OMAP_Module/131(OMAPve_g_ADAS_OBJ01_LgtDis) -> OMAPve_g_ADAS_OBJ01_LgtDis/1
  EWWWve_y_BSD_M_ErrorSt/1 -> OMAP_Module/101(EWWWve_y_BSD_M_ErrorSt)
  AEBSve_d_AEBFaultStatus/1 -> OMAP_Module/40(AEBSve_d_AEBFaultStatus)
  OMAP_Module/126(OMAPve_g_ADAS_R0_C0_COEF) -> OMAPve_g_ADAS_R0_C0_COEF/1
  OMAP_Module/83(OMAPve_y_ADAS_BSD_DOWWorkingSt) -> OMAPve_y_ADAS_BSD_DOWWorkingSt/1
  OMAP_Module/130(OMAPve_g_ADAS_OBJ01_LatDis) -> OMAPve_g_ADAS_OBJ01_LatDis/1
  OMAP_Module/97(OMAPve_y_ADAS_SRR_RF_SystStInfo) -> OMAPve_y_ADAS_SRR_RF_SystStInfo/1
  OMAP_Module/15(OMAPve_y_ADAS_AEBAlertReq) -> OMAPve_y_ADAS_AEBAlertReq/1
  OMAP_Module/75(OMAPve_y_ADAS_LeftLEDWarningSt) -> OMAPve_y_ADAS_LeftLEDWarningSt/1
  OMAP_Module/43(OMAPve_y_ADAS_LKAMode) -> OMAPve_y_ADAS_LKAMode/1
  OMAP_Module/123(OMAPve_g_ADAS_L0_C2_COEF) -> OMAPve_g_ADAS_L0_C2_COEF/1
  ACCSve_d_ACC_TqFlag/1 -> OMAP_Module/15(ACCSve_d_ACC_TqFlag)
  OMAP_Module/125(OMAPve_y_ADAS_R0_LINE_TYPE) -> OMAPve_y_ADAS_R0_LINE_TYPE/1
  OMAP_Module/107(OMAPve_y_ADAS_FrontObj01Class) -> OMAPve_y_ADAS_FrontObj01Class/1
  AEBSve_d_AEBSwitchStatus/1 -> OMAP_Module/39(AEBSve_d_AEBSwitchStatus)
  OMAP_Module/153(OMAPve_y_ADAS_OBJ05_ID) -> OMAPve_y_ADAS_OBJ05_ID/1
  JABSve_d_DbSignalTStamp/1 -> OMAP_Module/57(JABSve_d_DbSignalTStamp)
  EWWWve_y_SRR_SystemState/1 -> OMAP_Module/112(EWWWve_y_SRR_SystemState)
  OMAP_Module/120(OMAPve_y_ADAS_L0_LINE_TYPE) -> OMAPve_y_ADAS_L0_LINE_TYPE/1
  OMAP_Module/4(OMAPve_y_ADAS_ISAStatus) -> OMAPve_y_ADAS_ISAStatus/1
  OMAP_Module/32(OMAPve_y_ADAS_ESCHoldReq) -> OMAPve_y_ADAS_ESCHoldReq/1
  OMAP_Module/100(OMAPve_y_ADAS_SRR_RF_FCTAWrn) -> OMAPve_y_ADAS_SRR_RF_FCTAWrn/1
  AEBSve_d_JABS_HapticAlarm/1 -> OMAP_Module/48(AEBSve_d_JABS_HapticAlarm)
  OMAP_Module/27(OMAPve_y_ADAS_ACCState) -> OMAPve_y_ADAS_ACCState/1
  OMAP_Module/29(OMAPve_y_ADAS_DeclControlReq) -> OMAPve_y_ADAS_DeclControlReq/1
  ELKSve_y_EPS_State_Control/1 -> OMAP_Module/81(ELKSve_y_EPS_State_Control)
  OMAP_Module/159(OMAPve_y_ADAS_OBJ06_Lane) -> OMAPve_y_ADAS_OBJ06_Lane/1
  LKASve_y_EPS_LKA_Control/1 -> OMAP_Module/75(LKASve_y_EPS_LKA_Control)
  EWWWve_y_LCW_M_SystemWorkingSt/1 -> OMAP_Module/98(EWWWve_y_LCW_M_SystemWorkingSt)
  OMAP_Module/3(OMAPve_y_ADAS_ISASignType) -> OMAPve_y_ADAS_ISASignType/1
  OMAP_Module/57(OMAPve_y_ADAS_ICAStatusIcon) -> OMAPve_y_ADAS_ICAStatusIcon/1
  FDMMve_d_LkaFcnConf/1 -> OMAP_Module/5(FDMMve_d_LkaFcnConf)
  JABSve_d_DbSwitchStatus/1 -> OMAP_Module/59(JABSve_d_DbSwitchStatus)
  OMAP_Module/71(OMAPve_y_ADAS_LetfLigthControl) -> OMAPve_y_ADAS_LetfLigthControl/1
  OMAP_Module/116(OMAPve_y_ADAS_FrontObject06Zone) -> OMAPve_y_ADAS_FrontObject06Zone/1
  OMAP_Module/136(OMAPve_g_ADAS_OBJ02_LgtDis) -> OMAPve_g_ADAS_OBJ02_LgtDis/1
  LKASve_y_LDW_Status_Display/1 -> OMAP_Module/66(LKASve_y_LDW_Status_Display)
  OMAP_Module/28(OMAPve_g_ADAS_DecelerationSet) -> OMAPve_g_ADAS_DecelerationSet/1
  OMAP_Module/93(OMAPve_y_ADAS_SRR_LF_SystStInfo) -> OMAPve_y_ADAS_SRR_LF_SystStInfo/1
  OMAP_Module/49(OMAPve_y_ADAS_LKAState) -> OMAPve_y_ADAS_LKAState/1
  JABSve_d_DbJACWStatus/1 -> OMAP_Module/58(JABSve_d_DbJACWStatus)
  OMAP_Module/81(OMAPve_y_ADAS_BSD_DoorOpenWrn) -> OMAPve_y_ADAS_BSD_DoorOpenWrn/1
  OMAP_Module/137(OMAPve_y_ADAS_OBJ02_Class) -> OMAPve_y_ADAS_OBJ02_Class/1
  OMAP_Module/51(OMAPve_g_ADAS_LKAAngleReq) -> OMAPve_g_ADAS_LKAAngleReq/1
  OMAP_Module/96(OMAPve_y_ADAS_SRR_LF_FCTAWrn) -> OMAPve_y_ADAS_SRR_LF_FCTAWrn/1
  OMAP_Module/26(OMAPve_y_ADAS_UpDownGearChange) -> OMAPve_y_ADAS_UpDownGearChange/1
  LKASve_y_LKA_Action_Indication/1 -> OMAP_Module/70(LKASve_y_LKA_Action_Indication)
  OMAP_Module/114(OMAPve_y_ADAS_FrontObject05Zone) -> OMAPve_y_ADAS_FrontObject05Zone/1
  AEBSve_d_AEBAlertReq/1 -> OMAP_Module/41(AEBSve_d_AEBAlertReq)
  EWWWve_y_SRR_LF_FCTAWorkingSt/1 -> OMAP_Module/108(EWWWve_y_SRR_LF_FCTAWorkingSt)
  OMAP_Module/23(OMAPve_g_ADAS_ACCTorqueReq) -> OMAPve_g_ADAS_ACCTorqueReq/1
  OMAP_Module/154(OMAPve_y_ADAS_OBJ05_Lane) -> OMAPve_y_ADAS_OBJ05_Lane/1
  FDMMve_d_EwFcnConf/1 -> OMAP_Module/10(FDMMve_d_EwFcnConf)
  ICABve_d_ICAMode/1 -> OMAP_Module/92(ICABve_d_ICAMode)
  EWWWve_y_BSD_SystemStateInfo/1 -> OMAP_Module/114(EWWWve_y_BSD_SystemStateInfo)
  OMAP_Module/128(OMAPve_g_ADAS_R0_C2_COEF) -> OMAPve_g_ADAS_R0_C2_COEF/1
  OMAP_Module/101(OMAPve_y_ADAS_L0LineType) -> OMAPve_y_ADAS_L0LineType/1
  OMAP_Module/92(OMAPve_y_ADAS_BSD_S_RCTAWorkSt) -> OMAPve_y_ADAS_BSD_S_RCTAWorkSt/1
  ACCSve_d_ACC_DecFlag/1 -> OMAP_Module/17(ACCSve_d_ACC_DecFlag)
  ICABve_g_SteerAngleCmd/1 -> OMAP_Module/91(ICABve_g_SteerAngleCmd)
  OMAP_Module/1(OMAPve_y_ADAS_TSRSignType) -> OMAPve_y_ADAS_TSRSignType/1
  LKASve_y_LKA_Status_Display/1 -> OMAP_Module/67(LKASve_y_LKA_Status_Display)
  ACCSve_d_SignalTStamp/1 -> OMAP_Module/23(ACCSve_d_SignalTStamp)
  LKASve_y_HMI_Popup_Status/1 -> OMAP_Module/71(LKASve_y_HMI_Popup_Status)
  OMAP_Module/77(OMAPve_y_ADAS_BSD_SystemStInfo) -> OMAPve_y_ADAS_BSD_SystemStInfo/1
  EWWWve_y_BSD_M_RCTAWarning/1 -> OMAP_Module/104(EWWWve_y_BSD_M_RCTAWarning)
  OMAP_Module/94(OMAPve_y_ADAS_SRR_LF_SystWorkSt) -> OMAPve_y_ADAS_SRR_LF_SystWorkSt/1
  LKASve_y_Hands_Off_Warning/1 -> OMAP_Module/69(LKASve_y_Hands_Off_Warning)
  OMAP_Module/46(OMAPve_y_ADAS_ELKSts) -> OMAPve_y_ADAS_ELKSts/1
  OMAP_Module/48(OMAPve_y_ADAS_LCAPopupMessage) -> OMAPve_y_ADAS_LCAPopupMessage/1
  LKASve_y_LDW_Flag/1 -> OMAP_Module/68(LKASve_y_LDW_Flag)
  OMAP_Module/55(OMAPve_y_ADAS_ESARequest) -> OMAPve_y_ADAS_ESARequest/1
  ELKSve_y_ELK_VehicleLaneDisp/1 -> OMAP_Module/85(ELKSve_y_ELK_VehicleLaneDisp)
  OMAP_Module/73(OMAPve_y_ADAS_LightControlValid) -> OMAPve_y_ADAS_LightControlValid/1
  IMAPve_g_R0_C2/1 -> OMAP_Module/128(IMAPve_g_R0_C2)
  IMAPve_g_ESC_LonAcc/1 -> OMAP_Module/118(IMAPve_g_ESC_LonAcc)
  ICADva_d_LCRecommend/1 -> OMAP_Module/96(ICADva_d_LCRecommend)
  JABSve_d_DbFltStatus/1 -> OMAP_Module/60(JABSve_d_DbFltStatus)
  OMAP_Module/64(OMAPve_y_ADAS_IHBC_HB_Req) -> OMAPve_y_ADAS_IHBC_HB_Req/1
  EWWWve_y_BSD_S_DoorOpenWarning/1 -> OMAP_Module/106(EWWWve_y_BSD_S_DoorOpenWarning)
  AEBSve_d_JABS_Tips/1 -> OMAP_Module/49(AEBSve_d_JABS_Tips)
  OMAP_Module/142(OMAPve_y_ADAS_OBJ03_Class) -> OMAPve_y_ADAS_OBJ03_Class/1
  LKASve_y_Vehicle_Lane_Display/1 -> OMAP_Module/65(LKASve_y_Vehicle_Lane_Display)
  OMAP_Module/102(OMAPve_y_ADAS_L1LineType) -> OMAPve_y_ADAS_L1LineType/1
  OMAP_Module/18(OMAPve_y_ADAS_AEBMassageDisp) -> OMAPve_y_ADAS_AEBMassageDisp/1
  OMAP_Module/89(OMAPve_y_ADAS_BSD_S_DoorOpenWrn) -> OMAPve_y_ADAS_BSD_S_DoorOpenWrn/1
  OMAP_Module/47(OMAPve_y_ADAS_LCAStatusDisplay) -> OMAPve_y_ADAS_LCAStatusDisplay/1
  OMAP_Module/67(OMAPve_y_ADAS_ACCRequestEPB) -> OMAPve_y_ADAS_ACCRequestEPB/1
  OMAP_Module/135(OMAPve_g_ADAS_OBJ02_LatDis) -> OMAPve_g_ADAS_OBJ02_LatDis/1
  OMAP_Module/61(OMAPve_y_ADAS_JAFaultSt) -> OMAPve_y_ADAS_JAFaultSt/1
  OMAP_Module/68(OMAPve_y_ADAS_EngStartReqForSTT) -> OMAPve_y_ADAS_EngStartReqForSTT/1
  OMAP_Module/38(OMAPve_y_ADAS_Handsoffwarning) -> OMAPve_y_ADAS_Handsoffwarning/1
  ACCSve_d_ACC_ESCDriveOff/1 -> OMAP_Module/25(ACCSve_d_ACC_ESCDriveOff)
  IMAPva_d_obj_id/1 -> OMAP_Module/119(IMAPva_d_obj_id)
  OMAP_Module/124(OMAPve_g_ADAS_L0_C3_COEF) -> OMAPve_g_ADAS_L0_C3_COEF/1
  OMAP_Module/59(OMAPve_y_ADAS_HWATurnOnIdctr) -> OMAPve_y_ADAS_HWATurnOnIdctr/1
  OMAP_Module/151(OMAPve_g_ADAS_OBJ05_LgtDis) -> OMAPve_g_ADAS_OBJ05_LgtDis/1
  OMAP_Module/95(OMAPve_y_ADAS_SRR_LF_ErrorSt) -> OMAPve_y_ADAS_SRR_LF_ErrorSt/1
  OMAP_Module/53(OMAPve_y_ADAS_ESAState) -> OMAPve_y_ADAS_ESAState/1
  IMAPve_g_R0_C0/1 -> OMAP_Module/126(IMAPve_g_R0_C0)
  EWWWve_y_BSD_M_LCAWarning/1 -> OMAP_Module/102(EWWWve_y_BSD_M_LCAWarning)
  OMAP_Module/87(OMAPve_y_ADAS_BSD_S_ErrorSt) -> OMAPve_y_ADAS_BSD_S_ErrorSt/1
  EWWWve_y_RCTA_M_SystemWorkingSt/1 -> OMAP_Module/99(EWWWve_y_RCTA_M_SystemWorkingSt)
  OMAP_Module/143(OMAPve_y_ADAS_OBJ03_ID) -> OMAPve_y_ADAS_OBJ03_ID/1
  ELKSve_y_ELK_Action_Indication/1 -> OMAP_Module/79(ELKSve_y_ELK_Action_Indication)
  OMAP_Module/7(OMAPve_y_ADAS_ISLCDriverRemind) -> OMAPve_y_ADAS_ISLCDriverRemind/1
  JABSve_d_DbMDDdecRequest/1 -> OMAP_Module/53(JABSve_d_DbMDDdecRequest)
  OMAP_Module/121(OMAPve_g_ADAS_L0_C0_COEF) -> OMAPve_g_ADAS_L0_C0_COEF/1
  FDMMve_d_AlcFcnConf/1 -> OMAP_Module/9(FDMMve_d_AlcFcnConf)
  OMAP_Module/54(OMAPve_g_ADAS_ESATorqueReq) -> OMAPve_g_ADAS_ESATorqueReq/1
  ELKSve_y_ELK_HapticAlarmReq/1 -> OMAP_Module/77(ELKSve_y_ELK_HapticAlarmReq)
  OMAP_Module/34(OMAPve_y_ADAS_AEBState) -> OMAPve_y_ADAS_AEBState/1
  ACCSve_d_ACC_go_request/1 -> OMAP_Module/20(ACCSve_d_ACC_go_request)
  ELKSve_g_ELK_SWA_Control/1 -> OMAP_Module/82(ELKSve_g_ELK_SWA_Control)
  IMAPve_g_R0_C1/1 -> OMAP_Module/127(IMAPve_g_R0_C1)
  OMAP_Module/109(OMAPve_y_ADAS_FrontObj02Class) -> OMAPve_y_ADAS_FrontObj02Class/1
  OMAP_Module/56(OMAPve_y_ADAS_ICAMassageDisp) -> OMAPve_y_ADAS_ICAMassageDisp/1
  EWWWve_y_SRR_RF_FCTAWarning/1 -> OMAP_Module/111(EWWWve_y_SRR_RF_FCTAWarning)
  JABSve_d_DbAlertReq/1 -> OMAP_Module/61(JABSve_d_DbAlertReq)
  JABSve_d_DbPrefillReq/1 -> OMAP_Module/50(JABSve_d_DbPrefillReq)
  FDMMve_d_AccFcnConf/1 -> OMAP_Module/7(FDMMve_d_AccFcnConf)
  OMAP_Module/21(OMAPve_y_ADAS_ACCLongiDist) -> OMAPve_y_ADAS_ACCLongiDist/1
  ELKSve_y_Hands_Off_Warning/1 -> OMAP_Module/78(ELKSve_y_Hands_Off_Warning)
  JABSve_d_DbHapticAlarm/1 -> OMAP_Module/55(JABSve_d_DbHapticAlarm)
  OMAP_Module/108(OMAPve_y_ADAS_FrontObject02Zone) -> OMAPve_y_ADAS_FrontObject02Zone/1
  AEBSve_d_AEBTips/1 -> OMAP_Module/42(AEBSve_d_AEBTips)
  OMAP_Module/86(OMAPve_y_ADAS_BSD_S_LCWWorkSt) -> OMAPve_y_ADAS_BSD_S_LCWWorkSt/1
  OMAP_Module/24(OMAPve_y_ADAS_TorqueActivReq) -> OMAPve_y_ADAS_TorqueActivReq/1
  OMAP_Module/41(OMAPve_y_ADAS_LDWWarningSt) -> OMAPve_y_ADAS_LDWWarningSt/1
  ELKSve_y_EPS_ELK_Control/1 -> OMAP_Module/84(ELKSve_y_EPS_ELK_Control)
  OMAP_Module/37(OMAPve_y_ADAS_HapticAlarmReq) -> OMAPve_y_ADAS_HapticAlarmReq/1
  OMAP_Module/5(OMAPve_y_ADAS_ISAValue) -> OMAPve_y_ADAS_ISAValue/1
  EWWWve_y_BSD_S_RCTAWarning/1 -> OMAP_Module/107(EWWWve_y_BSD_S_RCTAWarning)
  OMAP_Module/157(OMAPve_y_ADAS_OBJ06_Class) -> OMAPve_y_ADAS_OBJ06_Class/1
  OMAP_Module/80(OMAPve_y_ADAS_BSD_LCAWarning) -> OMAPve_y_ADAS_BSD_LCAWarning/1
  OMAP_Module/20(OMAPve_y_ADAS_TargetPosition) -> OMAPve_y_ADAS_TargetPosition/1
  ACCSve_d_ACC_ICA_Flag/1 -> OMAP_Module/24(ACCSve_d_ACC_ICA_Flag)
  ACCSve_g_ACC_TqReq/1 -> OMAP_Module/14(ACCSve_g_ACC_TqReq)
  AEBSve_d_HapticAlarm/1 -> OMAP_Module/35(AEBSve_d_HapticAlarm)
  OMAP_Module/150(OMAPve_g_ADAS_OBJ05_LatDis) -> OMAPve_g_ADAS_OBJ05_LatDis/1
  EWWWve_y_BSD_S_SystemStateInfo/1 -> OMAP_Module/113(EWWWve_y_BSD_S_SystemStateInfo)
  OMAP_Module/39(OMAPve_y_ADAS_HMIPopupMassage) -> OMAPve_y_ADAS_HMIPopupMassage/1
  JABSve_g_DbDecSetpoint/1 -> OMAP_Module/52(JABSve_g_DbDecSetpoint)
  OMAP_Module/60(OMAPve_y_ADAS_ESAFaultSt) -> OMAPve_y_ADAS_ESAFaultSt/1
  OMAP_Module/115(OMAPve_y_ADAS_FrontObj05Class) -> OMAPve_y_ADAS_FrontObj05Class/1
  FDMMve_d_LfFcnConf/1 -> OMAP_Module/8(FDMMve_d_LfFcnConf)
  OMAP_Module/17(OMAPve_y_ADAS_AEBSwitchStatus) -> OMAPve_y_ADAS_AEBSwitchStatus/1
  OMAP_Module/133(OMAPve_y_ADAS_OBJ01_ID) -> OMAPve_y_ADAS_OBJ01_ID/1
  JABSve_d_DbFunFARCSta/1 -> OMAP_Module/51(JABSve_d_DbFunFARCSta)
  AEBSve_d_functionFARCState/1 -> OMAP_Module/29(AEBSve_d_functionFARCState)
  OMAP_Module/14(OMAPve_y_ADAS_ACCMessagePrompt) -> OMAPve_y_ADAS_ACCMessagePrompt/1
  JABSve_d_DbTips/1 -> OMAP_Module/62(JABSve_d_DbTips)
  ELKSve_g_EPS_Factor_Control/1 -> OMAP_Module/83(ELKSve_g_EPS_Factor_Control)
  OMAP_Module/76(OMAPve_y_ADAS_RighrLEDWarningSt) -> OMAPve_y_ADAS_RighrLEDWarningSt/1
  AEBSve_d_JABS_AlertSign/1 -> OMAP_Module/44(AEBSve_d_JABS_AlertSign)
  OMAP_Module/112(OMAPve_y_ADAS_FrontObject04Zone) -> OMAPve_y_ADAS_FrontObject04Zone/1
  OMAP_Module/91(OMAPve_y_ADAS_BSD_S_DOWWorkSt) -> OMAPve_y_ADAS_BSD_S_DOWWorkSt/1
  OMAP_Module/13(OMAPve_y_ADAS_ACC_RVVReqType) -> OMAPve_y_ADAS_ACC_RVVReqType/1
  AEBSve_d_MDDdecType/1 -> OMAP_Module/32(AEBSve_d_MDDdecType)
  JABSve_d_DbESCHoldReq/1 -> OMAP_Module/64(JABSve_d_DbESCHoldReq)
  OMAP_Module/138(OMAPve_y_ADAS_OBJ02_ID) -> OMAPve_y_ADAS_OBJ02_ID/1
  AEBSve_d_SignalTStamp/1 -> OMAP_Module/43(AEBSve_d_SignalTStamp)
  OMAP_Module/19(OMAPve_y_ADAS_HMITargetDispFlag) -> OMAPve_y_ADAS_HMITargetDispFlag/1
  OMAP_Module/106(OMAPve_y_ADAS_FrontObject01Zone) -> OMAPve_y_ADAS_FrontObject01Zone/1
  EWWWve_y_SRR_LF_SystemStateInfo/1 -> OMAP_Module/115(EWWWve_y_SRR_LF_SystemStateInfo)
  ICADva_d_DecionCMD/1 -> OMAP_Module/95(ICADva_d_DecionCMD)
  EWWWve_y_BSD_M_DoorOpenWarning/1 -> OMAP_Module/103(EWWWve_y_BSD_M_DoorOpenWarning)
  OMAP_Module/16(OMAPve_y_ADAS_AEBFaultStatus) -> OMAPve_y_ADAS_AEBFaultStatus/1
  OMAP_Module/22(OMAPve_y_ADAS_ACCLateralDist) -> OMAPve_y_ADAS_ACCLateralDist/1
  AEBSve_d_Prefill_request/1 -> OMAP_Module/28(AEBSve_d_Prefill_request)
  OMAP_Module/88(OMAPve_y_ADAS_BSD_S_LCAWarning) -> OMAPve_y_ADAS_BSD_S_LCAWarning/1
  ELKSve_y_ELK_ELKSts/1 -> OMAP_Module/86(ELKSve_y_ELK_ELKSts)
  OMAP_Module/62(OMAPve_y_ADAS_HWAActionSts) -> OMAPve_y_ADAS_HWAActionSts/1
  AEBSve_d_AEBStatus/1 -> OMAP_Module/37(AEBSve_d_AEBStatus)
  ELKSve_y_state_ELK_function/1 -> OMAP_Module/76(ELKSve_y_state_ELK_function)
  IMAPve_d_ESC_Veh_Standstill/1 -> OMAP_Module/121(IMAPve_d_ESC_Veh_Standstill)
  OMAP_Module/129(OMAPve_g_ADAS_R0_C3_COEF) -> OMAPve_g_ADAS_R0_C3_COEF/1
  ACCSve_g_ACC_DecReq/1 -> OMAP_Module/16(ACCSve_g_ACC_DecReq)
  OMAP_Module/139(OMAPve_y_ADAS_OBJ02_Lane) -> OMAPve_y_ADAS_OBJ02_Lane/1
  OMAP_Module/98(OMAPve_y_ADAS_SRR_RF_SystWorkSt) -> OMAPve_y_ADAS_SRR_RF_SystWorkSt/1
  OMAP_Module/144(OMAPve_y_ADAS_OBJ03_Lane) -> OMAPve_y_ADAS_OBJ03_Lane/1
  EWWWve_y_SRR_LF_FCTAWarning/1 -> OMAP_Module/110(EWWWve_y_SRR_LF_FCTAWarning)
  OMAP_Module/40(OMAPve_y_ADAS_VehicleLaneDisp) -> OMAPve_y_ADAS_VehicleLaneDisp/1
  AEBSve_d_MDDdecRequest/1 -> OMAP_Module/31(AEBSve_d_MDDdecRequest)
  LKASve_y_EPS_State_Control/1 -> OMAP_Module/72(LKASve_y_EPS_State_Control)
  OMAP_Module/12(OMAPve_y_ADAS_ACCStatusIconDis) -> OMAPve_y_ADAS_ACCStatusIconDis/1
  OMAP_Module/11(OMAPve_y_ADAS_ACCSetSpeedDis) -> OMAPve_y_ADAS_ACCSetSpeedDis/1
  OMAP_Module/35(OMAPve_y_ADAS_BrakeRequest) -> OMAPve_y_ADAS_BrakeRequest/1
  OMAP_Module/149(OMAPve_y_ADAS_OBJ04_Lane) -> OMAPve_y_ADAS_OBJ04_Lane/1
  ACCSve_d_ACCActive_Signal/1 -> OMAP_Module/19(ACCSve_d_ACCActive_Signal)
  OMAP_Module/9(OMAPve_y_ADAS_ACCHeadwayIcon) -> OMAPve_y_ADAS_ACCHeadwayIcon/1
  OMAP_Module/10(OMAPve_y_ADAS_ACCSetSpeed) -> OMAPve_y_ADAS_ACCSetSpeed/1
  LKASve_g_EPS_Factor_Control/1 -> OMAP_Module/74(LKASve_g_EPS_Factor_Control)
  AEBSve_d_JABS_FltStatus/1 -> OMAP_Module/46(AEBSve_d_JABS_FltStatus)
  OMAP_Module/146(OMAPve_g_ADAS_OBJ04_LgtDis) -> OMAPve_g_ADAS_OBJ04_LgtDis/1
  ICABve_d_SignalTStamp/1 -> OMAP_Module/89(ICABve_d_SignalTStamp)
  ICABva_d_ICAB2HMI/1 -> OMAP_Module/90(ICABva_d_ICAB2HMI)
  OMAP_Module/45(OMAPve_y_ADAS_LKASwitchState) -> OMAPve_y_ADAS_LKASwitchState/1
  ICADve_d_SignalTStamp/1 -> OMAP_Module/97(ICADve_d_SignalTStamp)
  OMAP_Module/147(OMAPve_y_ADAS_OBJ04_Class) -> OMAPve_y_ADAS_OBJ04_Class/1
  FDMMve_g_Adas2Fapa/1 -> OMAP_Module/11(FDMMve_g_Adas2Fapa)
  AEBSve_d_ESCHoldReq/1 -> OMAP_Module/34(AEBSve_d_ESCHoldReq)
  FDMMve_d_AebFcnConf/1 -> OMAP_Module/2(FDMMve_d_AebFcnConf)
  ELKSve_y_HMI_Popup_Status/1 -> OMAP_Module/80(ELKSve_y_HMI_Popup_Status)
  AEBSve_d_Braking_progress/1 -> OMAP_Module/36(AEBSve_d_Braking_progress)
  OMAP_Module/74(OMAPve_y_ADAS_SRR_SystemState) -> OMAPve_y_ADAS_SRR_SystemState/1
  OMAP_Module/50(OMAPve_g_ADAS_LKATorqFactReq) -> OMAPve_g_ADAS_LKATorqFactReq/1
  OMAP_Module/25(OMAPve_g_ADAS_DownorUpGearMinTime) -> OMAPve_g_ADAS_DownorUpGearMinTime/1
  OMAP_Module/52(OMAPve_y_ADAS_LKAActivation) -> OMAPve_y_ADAS_LKAActivation/1
  OMAP_Module/103(OMAPve_y_ADAS_R0LineType) -> OMAPve_y_ADAS_R0LineType/1
  OMAP_Module/30(OMAPve_y_ADAS_PrefillRequest) -> OMAPve_y_ADAS_PrefillRequest/1
